simulink library "RifftLib"  (R2022b)
settings: Solver=VariableStepAuto  StartTime=0.0  StopTime=10.0  RelTol=1e-3
undefined symbols (not defined in the file or in its folder): RifftTestSettings
libraries: HandyTextFile x6, ITC x2
settings Model: Creator=ud1041536  LastModifiedBy=fz1054048
settings SolverCC: AlgebraicLoopSolver=TrustRegion
settings DebuggingCC: UnconnectedInputMsg=warning  UnconnectedOutputMsg=warning  UnconnectedLineMsg=warning  SFMachineParentedDataDiag=warning  ArithmeticOperatorsInVariantConditions=warning
settings ModelReferenceCC: EnableRefExpFcnMdlSchedulingChecks=on
settings SFSimCC: CustomCodeUndefinedFunction=UseInterfaceOnly
settings RTWCC: DLArmComputeVersion=19.05

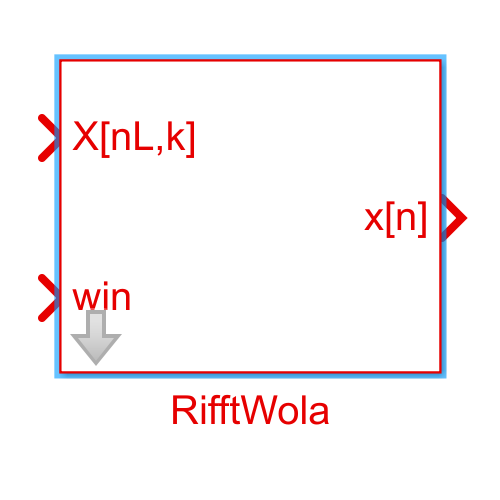
[thumbnail: Simulink's stored preview of the top-level diagram]
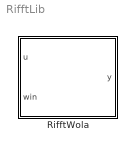
== system RifftLib ==
  RifftWola : Subsystem  mask(Blocklib Rifft){Config=RifftTestSettings.Rifft}
      mask prompts: Config "RifftWolaConfig"
      mask help:
      | See 'Help' or run
      | >> help RifftWolaConfig
      mask init:
      | blkh=gcbh;
      | Config=BTConfig.Assert(blkh,Config);
      | 
      | Config.Validate();
      | Config.DoMaskInit(blkh);
      mask Help: eval('help RifftWolaConfig')
      mask Display:
      | port_label('output',1,'x[n]')
      | port_label('input',1,'X[nL,k]')
      | port_label('input',2,'win')

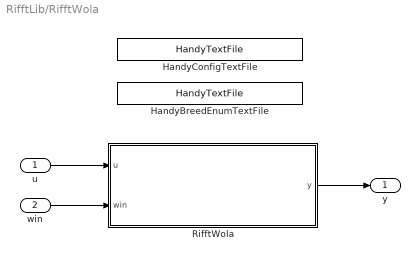
== system RifftLib/RifftWola ==
  u : Inport
  win : Inport  Port=2
  HandyBreedEnumTextFile : HandyTextFile/HandyTextFile  TemplateSource=<dialog fields>  FileSuffix=BreedEnum  OpenDialogOnLoad=off  UseThisBlockName=off  AddGrandParentNamePrefix=off  TheDefaultText=% $(FILENAME) $(PREFIX) $(SUFFIX)  ShowInLibBrowser=on
      settings: SourceProductName=Bose Talaria
  HandyConfigTextFile : HandyTextFile/HandyTextFile  TemplateSource=Config  FileSuffix=File  OpenDialogOnLoad=off  UseThisBlockName=off  AddGrandParentNamePrefix=off  TheDefaultText=% $(FILENAME) $(PREFIX) $(SUFFIX)  ShowInLibBrowser=on
      settings: SourceProductName=Bose Talaria
  RifftWola : Subsystem  Variant=on
  y : Outport  VectorParamsAs1DForOutWhenUnconnected=off
  wires:
  RifftWola/1(y) -> y/1
  u/1 -> RifftWola/1(u)
  win/1 -> RifftWola/2(win)

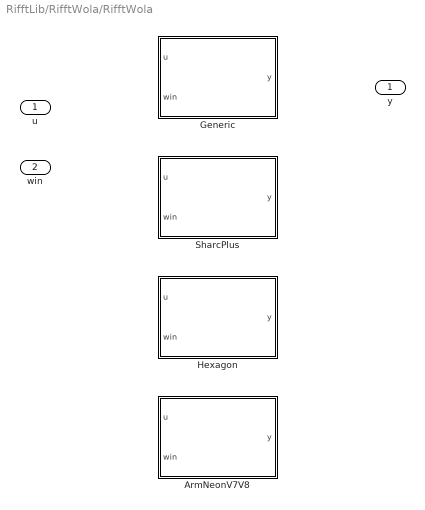
== system RifftLib/RifftWola/RifftWola ==
  u : Inport
  win : Inport  Port=2
  ArmNeonV7V8 : Subsystem  VariantControl=Config.Breed == AsdHwEnum.ArmNeonV7V8
  Generic : Subsystem  VariantControl=(default)
  Hexagon : Subsystem  VariantControl=Config.Breed == AsdHwEnum.Hexagon
  SharcPlus : Subsystem  VariantControl=Config.Breed == AsdHwEnum.SharcPlus
  y : Outport

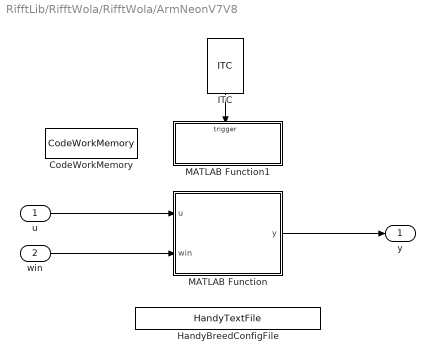
== system RifftLib/RifftWola/RifftWola/ArmNeonV7V8 ==
  u : Inport
  win : Inport  Port=2
  CodeWorkMemory : DataStoreMemory  DataStoreName=CodeWorkMemory  WriteAfterWriteMsg=warning  InitialValue=Config.BreedObj.DsmCodeWorkMemoryInitValue  ShowAdditionalParam=off  OutDataTypeStr=uint32
  HandyBreedConfigFile : HandyTextFile/HandyTextFile  TemplateSource=<dialog fields>  FileSuffix=BreedEnum  OpenDialogOnLoad=off  UseThisBlockName=off  AddGrandParentNamePrefix=on  TheDefaultText=|  ShowInLibBrowser=on
      | % $(FILENAME) Setup model parameters for each "Init" callback (e.g. update diagram)
      | sample_rate_in_hertz = 44100;
      | frame_size = 32;
      | sysin_channel_count = 2;
      settings: SourceProductName=Bose Talaria
  ITC : ITC/ITC
      settings: SourceProductName=Bose Talaria
  MATLAB Function : MATLAB Function  TreatAsAtomicUnit=on  mask{fftSize=Config.FftSize, numOverlap=Config.NumOverlap}
  MATLAB Function1 : MATLAB Function  TreatAsAtomicUnit=on  mask{fftSize=Config.FftSize}
  y : Outport
  wires:
  u/1 -> MATLAB Function/1(u)
  win/1 -> MATLAB Function/2(win)
  MATLAB Function/1(y) -> y/1
  ITC/1 -> MATLAB Function1/Trigger

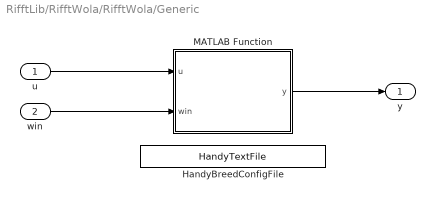
== system RifftLib/RifftWola/RifftWola/Generic ==
  u : Inport
  win : Inport  Port=2
  HandyBreedConfigFile : HandyTextFile/HandyTextFile  TemplateSource=<dialog fields>  FileSuffix=BreedEnum  OpenDialogOnLoad=off  UseThisBlockName=off  AddGrandParentNamePrefix=on  TheDefaultText=|  ShowInLibBrowser=on
      | % $(FILENAME) Setup model parameters for each "Init" callback (e.g. update diagram)
      | sample_rate_in_hertz = 44100;
      | frame_size = 32;
      | sysin_channel_count = 2;
      settings: SourceProductName=Bose Talaria
  MATLAB Function : MATLAB Function  TreatAsAtomicUnit=on  mask{fftSize=Config.FftSize, numOverlap=Config.NumOverlap}
  y : Outport
  wires:
  u/1 -> MATLAB Function/1(u)
  win/1 -> MATLAB Function/2(win)
  MATLAB Function/1(y) -> y/1

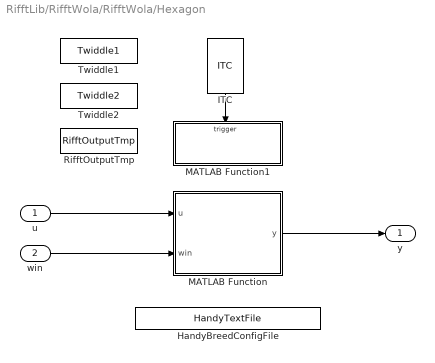
== system RifftLib/RifftWola/RifftWola/Hexagon ==
  u : Inport
  win : Inport  Port=2
  HandyBreedConfigFile : HandyTextFile/HandyTextFile  TemplateSource=<dialog fields>  FileSuffix=BreedEnum  OpenDialogOnLoad=off  UseThisBlockName=off  AddGrandParentNamePrefix=on  TheDefaultText=|  ShowInLibBrowser=on
      | % $(FILENAME) Setup model parameters for each "Init" callback (e.g. update diagram)
      | sample_rate_in_hertz = 44100;
      | frame_size = 32;
      | sysin_channel_count = 2;
      settings: SourceProductName=Bose Talaria
  ITC : ITC/ITC
      settings: SourceProductName=Bose Talaria
  MATLAB Function : MATLAB Function  TreatAsAtomicUnit=on  mask{fftSize=Config.FftSize, numOverlap=Config.NumOverlap}
  MATLAB Function1 : MATLAB Function  TreatAsAtomicUnit=on  mask{fftSize=Config.FftSize}
  RifftOutputTmp : DataStoreMemory  DataStoreName=RifftOutputTmp  WriteAfterWriteMsg=warning  InitialValue=Config.BreedObj.DsmRifftOutputTmpInitValue  ShowAdditionalParam=off  OutDataTypeStr=single
      settings: SignalType=complex
  Twiddle1 : DataStoreMemory  DataStoreName=Twiddle1  WriteAfterWriteMsg=warning  InitialValue=Config.BreedObj.DsmTwiddle1InitValue  ShowAdditionalParam=off  OutDataTypeStr=single
      settings: SignalType=complex
  Twiddle2 : DataStoreMemory  DataStoreName=Twiddle2  WriteAfterWriteMsg=warning  InitialValue=Config.BreedObj.DsmTwiddle2InitValue  ShowAdditionalParam=off  OutDataTypeStr=single
      settings: SignalType=complex
  y : Outport
  wires:
  u/1 -> MATLAB Function/1(u)
  win/1 -> MATLAB Function/2(win)
  MATLAB Function/1(y) -> y/1
  ITC/1 -> MATLAB Function1/Trigger

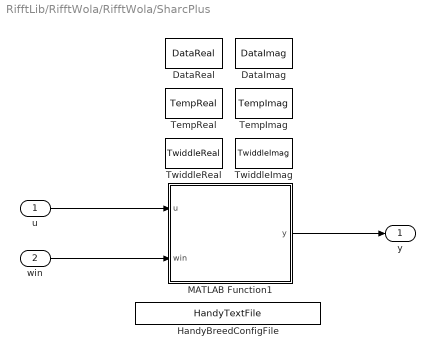
== system RifftLib/RifftWola/RifftWola/SharcPlus ==
  u : Inport
  win : Inport  Port=2
  DataImag : DataStoreMemory  DataStoreName=DataImag  ReadBeforeWriteMsg=warning  WriteAfterWriteMsg=warning  WriteAfterReadMsg=warning  InitialValue=Config.BreedObj.DsmDataImagInitValue  ShowAdditionalParam=off  OutDataTypeStr=single
  DataReal : DataStoreMemory  DataStoreName=DataReal  ReadBeforeWriteMsg=warning  WriteAfterWriteMsg=warning  WriteAfterReadMsg=warning  InitialValue=Config.BreedObj.DsmDataRealInitValue  ShowAdditionalParam=off  OutDataTypeStr=single
  HandyBreedConfigFile : HandyTextFile/HandyTextFile  TemplateSource=<dialog fields>  FileSuffix=BreedEnum  OpenDialogOnLoad=off  UseThisBlockName=off  AddGrandParentNamePrefix=on  TheDefaultText=|  ShowInLibBrowser=on
      | % $(FILENAME) Setup model parameters for each "Init" callback (e.g. update diagram)
      | sample_rate_in_hertz = 44100;
      | frame_size = 32;
      | sysin_channel_count = 2;
      settings: SourceProductName=Bose Talaria
  MATLAB Function1 : MATLAB Function  TreatAsAtomicUnit=on  mask{fftSize=Config.FftSize, numOverlap=Config.NumOverlap}
  TempImag : DataStoreMemory  DataStoreName=TempImag  ReadBeforeWriteMsg=warning  WriteAfterWriteMsg=warning  WriteAfterReadMsg=warning  InitialValue=Config.BreedObj.DsmTempImagInitValue  ShowAdditionalParam=off  OutDataTypeStr=single
  TempReal : DataStoreMemory  DataStoreName=TempReal  ReadBeforeWriteMsg=warning  WriteAfterWriteMsg=warning  WriteAfterReadMsg=warning  InitialValue=Config.BreedObj.DsmTempRealInitValue  ShowAdditionalParam=off  OutDataTypeStr=single
  TwiddleImag : DataStoreMemory  DataStoreName=TwiddleImag  ReadBeforeWriteMsg=warning  WriteAfterWriteMsg=warning  WriteAfterReadMsg=warning  InitialValue=Config.BreedObj.DsmTwiddleImagInitValue  ShowAdditionalParam=off  OutDataTypeStr=uint32
  TwiddleReal : DataStoreMemory  DataStoreName=TwiddleReal  ReadBeforeWriteMsg=warning  WriteAfterWriteMsg=warning  WriteAfterReadMsg=warning  InitialValue=Config.BreedObj.DsmTwiddleRealInitValue  ShowAdditionalParam=off  OutDataTypeStr=uint32
  y : Outport
  wires:
  u/1 -> MATLAB Function1/1(u)
  win/1 -> MATLAB Function1/2(win)
  MATLAB Function1/1(y) -> y/1

== matlab function RifftLib/RifftWola/RifftWola/ArmNeonV7V8/MATLAB Function ==
  data: u input; y output; win input; fftSize parameter; numOverlap parameter; CodeWorkMemory data_store_memory
function y = Rifft(u, win, fftSize, numOverlap)

global CodeWorkMemory;

[~, numChannels] = size(u);
outputSize = fftSize - numOverlap;

% Buffer to hold overlapped samples
persistent outputOverlap;
if isempty(outputOverlap)
    outputOverlap = single(zeros(numOverlap, numChannels));
end

% Buffer for Simulation 
persistent lastFrame;

% Nullcopy copies type, size, and complexity of input to output
y = coder.nullcopy(single(zeros(outputSize, numChannels)));

% Simulation
if(coder.target('MATLAB') || coder.target('Sfun')) 
  % Buffer to hold overlapped samples
    numChannels = size(u,2);
    if isempty(lastFrame)
        lastFrame = single(zeros(numOverlap, numChannels));
    end
    [y, lastFrame] = RifftProcessSim(u, win, numOverlap, lastFrame);

% Code generation
else
    y = rifft_armv7v8_process(complex(single(u)), uint32(numChannels), uint32(fftSize), uint32(numOverlap), ...
                       single(win), single(outputOverlap), uint32(CodeWorkMemory));
    % NOTE: The CRL mechanism requires an output for the function call,
    % and appears to be optimized out if that return value isn't used. 
    % This is a dummy operation to make sure CRL ends up in generated code    
end
end
 

%% CRL function for code generation
function y = rifft_armv7v8_process(u, num_ch, fft_size, num_overlap, win, output_overlap, codeworkmemory)
% If target == codegen, error out if no CRL found
coder.replace('-errorifnoreplacement'); 
y = (single(zeros(fft_size - num_overlap, num_ch)));
end

== matlab function RifftLib/RifftWola/RifftWola/Hexagon/MATLAB Function ==
  data: u input; y output; win input; fftSize parameter; Twiddle1 data_store_memory; Twiddle2 data_store_memory; RifftOutputTmp data_store_memory; numOverlap parameter
function y = Rifft(u, win, fftSize, numOverlap)

global Twiddle1;
global Twiddle2;
global RifftOutputTmp;

[~, numChannels] = size(u);
outputSize = fftSize - numOverlap;

% Buffer to hold overlapped samples
persistent outputOverlap;
if isempty(outputOverlap)
    outputOverlap = single(zeros(numOverlap, numChannels));
end

% Buffer for Simulation 
persistent lastFrame;

% Nullcopy copies type, size, and complexity of input to output
y = coder.nullcopy(single(zeros(outputSize, numChannels)));

% Simulation
if(coder.target('MATLAB') || coder.target('Sfun')) 
  % Buffer to hold overlapped samples
    numChannels = size(u,2);
    if isempty(lastFrame)
        lastFrame = single(zeros(numOverlap, numChannels));
    end
    [y, lastFrame] = RifftProcessSim(u, win, numOverlap, lastFrame);


% Code generation
else
   y = rifft_process(   single(complex(u)), ...
                        single(Twiddle1),...
                        single(Twiddle2),... 
                        single(RifftOutputTmp),...
                        single(win),...
                        outputOverlap,...
                        int32(fftSize),...
                        int32(numChannels),...
                        int32(numOverlap));
end

end

%% CRL function for code generation
function y = rifft_process( u,...
                            Twiddle1,...
                            Twiddle2,...
                            RifftOutputTmp,...
                            win,...                            
                            outputOverlap,...
                            fftSize,...
                            numChannels,...
                            numOverlap)
% If target == codegen, error out if no CRL found
coder.replace('-errorifnoreplacement');
y = single(zeros(fftSize - numOverlap, numChannels));
end

== matlab function RifftLib/RifftWola/RifftWola/Generic/MATLAB Function ==
  data: u input; y output; win input; fftSize parameter; numOverlap parameter
 function y = Rifft(u, win, fftSize, numOverlap)

% Buffer to hold overlapped samples
numChannels = size(u,2);
persistent lastFrame;
if isempty(lastFrame)
    lastFrame = single(zeros(numOverlap, numChannels));
end
[y, lastFrame] = RifftProcessSim(u, win, numOverlap, lastFrame);

end

== matlab function RifftLib/RifftWola/RifftWola/ArmNeonV7V8/MATLAB Function1 ==
  data: fftSize parameter; CodeWorkMemory data_store_memory
  events: trigger input FUNCTION_CALL_EVENT
function RifftInit(fftSize)

global CodeWorkMemory;

if ~(coder.target('MATLAB') || coder.target('Sfun')) 
    y = rfft_armv7v8_init(uint32(fftSize), uint32(CodeWorkMemory));    
    % NOTE: The CRL mechanism requires an output for the function call,
    % and appears to be optimized out if that return value isn't used. 
    % This is a dummy operation to make sure CRL ends up in generated code    
    CodeWorkMemory(1) = y;
end
end

function y = rfft_armv7v8_init(fftSize, workMemory)
% If target == codegen, error out if no CRL found
coder.replace('-errorifnoreplacement');
% No init simulation code, but need to do something to ensure CRL does not
% get optimized out
y = uint32(workMemory(1)) + fftSize;
end

== matlab function RifftLib/RifftWola/RifftWola/Hexagon/MATLAB Function1 ==
  data: fftSize parameter; Twiddle1 data_store_memory; Twiddle2 data_store_memory
  events: trigger input FUNCTION_CALL_EVENT
function RifftInit(fftSize)
% Initializes the Twiddle factors used for RFFT computation

global Twiddle1;
global Twiddle2;

% Intialize Twiddle Factors
[Twiddle1, Twiddle2] = rfft_init(int32(fftSize));

end

function [Twiddle1, Twiddle2] = rfft_init(fftSize)
% Twiddle1: Twiddle factor for N/2-point complex FFT
% Twiddle2: Twiddle factors for last stage
% If target == codegen, error out if no CRL found
coder.replace('-errorifnoreplacement');
Twiddle1 = single(complex(zeros(3*fftSize/8,1)));
Twiddle2 = single(complex(zeros(fftSize/2,1)));

end

== matlab function RifftLib/RifftWola/RifftWola/SharcPlus/MATLAB Function1 ==
  data: u input; win input; y output; fftSize parameter; numOverlap parameter; DataReal data_store_memory; DataImag data_store_memory; TempReal data_store_memory; TempImag data_store_memory; TwiddleReal data_store_memory; TwiddleImag data_store_memory
 function y = Rifft(u, win, fftSize, numOverlap)   

global DataReal
global DataImag
global TempReal
global TempImag
global TwiddleReal
global TwiddleImag

[~, numChannels] = size(u);
outputSize = fftSize - numOverlap;

% Buffer to hold overlapped samples
persistent outputOverlap;
if isempty(outputOverlap)
    outputOverlap = single(zeros(numOverlap, numChannels));
end

% Buffer for Simulation
persistent lastFrame;

% Nullcopy copies type, size, and complexity of input to output
y = coder.nullcopy(single(zeros(outputSize, numChannels)));

% Set correct data types
fftSize = uint32(fftSize);
numChannels = uint32(numChannels);
numOverlap = uint32(numOverlap);

% Simulation
if(coder.target('MATLAB') || coder.target('Sfun')) 
   % Buffer to hold overlapped samples
    numChannels = size(u,2);
    if isempty(lastFrame)
        lastFrame = single(zeros(numOverlap, numChannels));
    end
    [y, lastFrame] = RifftProcessSim(u, win, numOverlap, lastFrame);
    
% Code generation
else
    % Set the twiddle pointers to correct twiddle table
    % The pointers are of type uint32 here and will be casted to float* 
    % in the code-replaced function. The twiddle tables are declared in 
    % a separate file and will be pulled in through CRL.
    if fftSize == 256
        coder.ceval('set_twiddle_256', coder.wref(TwiddleReal), coder.wref(TwiddleImag));
    else
        coder.ceval('set_twiddle_128', coder.wref(TwiddleReal), coder.wref(TwiddleImag));
    end
    y = rifft_process(complex(single(u)), DataReal, DataImag, TempReal, TempImag, single(win), ...
        outputOverlap, TwiddleReal, TwiddleImag, fftSize, numChannels, numOverlap);
        
end

end    

%% CRL function for code generation
function y = rifft_process(u, data_r, data_i, temp_r, temp_i, win, ...
    output_overlap, twiddle_r, twiddle_i, fft_size, num_channel, num_overlap)
% If target == codegen, error out if no CRL found
coder.replace('-errorifnoreplacement'); 
y = (single(zeros(fft_size - num_overlap, num_channel)));

end
